simulink model "untitled1"  (R2022a)
settings: Solver=FixedStepAuto  StartTime=0.0  StopTime=10.0  RelTol=1e-3  EnableMultiTasking=on
settings Model: ExtModeTrigDuration=2  Creator=Asus  LastModifiedBy=Asus
settings OptimizationCC: EnhancedBackFolding=on  PassReuseOutputArgsAs=Individual arguments  ZeroExternalMemoryAtStartup=off  ZeroInternalMemoryAtStartup=off  MaxStackSize=64  OptimizeBlockOrder=speed  DifferentSizesBufferReuse=on  OptimizationCustomize=off  EfficientTunableParamExpr=on
settings DebuggingCC: ParameterTunabilityLossMsg=error
settings HardwareCC: ProdBitPerInt=16  ProdBitPerPointer=16  ProdBitPerSizeT=16  ProdBitPerPtrDiffT=16  ProdLargestAtomicFloat=None  ProdWordSize=8  ProdHWDeviceType=Atmel->AVR
settings SFSimCC: MATLABDynamicMemAlloc=off
settings RTWCC: SystemTargetFile=ert.tlc  HardwareBoard=Arduino Mega 2560  TemplateMakefile=ert_default_tmf  GenerateReport=on  Toolchain=Arduino AVR  BuildConfiguration=Faster Runs  LaunchReport=on
settings CodeAppCC: ForceParamTrailComments=on  IgnoreCustomStorageClasses=off  OperatorAnnotations=on  SimulinkDataObjDesc=on  SFDataObjDesc=on  InsertBlockDesc=on
settings ERTTargetCC: SupportContinuousTime=on  SupportVariableSizeSignals=on  ExtModeTransport=3  ExtModeStaticAlloc=on  ExtModeStaticAllocSize=2048  ExtModeMexFile=ext_xcp  ExtModeIntrfLevel=Level2 - Open

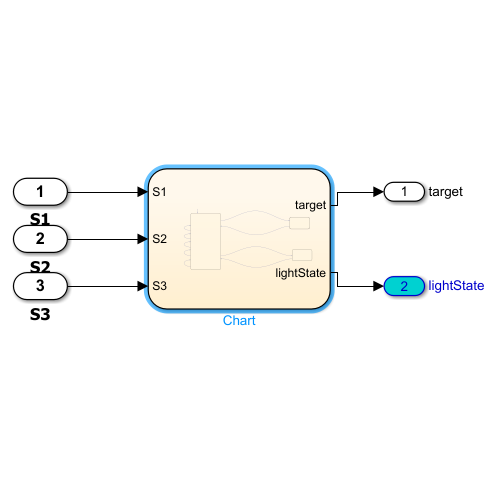
[thumbnail: Simulink's stored preview of the top-level diagram]
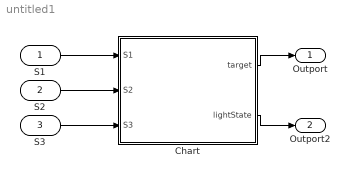
== system untitled1 ==
  S1 : Inport  OutDataTypeStr=boolean
  S2 : Inport  Port=2  OutDataTypeStr=boolean
  S3 : Inport  Port=3  OutDataTypeStr=boolean
  Chart : Stateflow chart  TreatAsAtomicUnit=on
  Outport : Outport  SignalName=target
  Outport2 : Outport  Port=2  SignalName=lightState
  wires:
  S2/1 -> Chart/2(S2)
  S3/1 -> Chart/3(S3)
  Chart/1(target) -> Outport/1
  Chart/2(lightState) -> Outport2/1
  S1/1 -> Chart/1(S1)

== stateflow chart untitled1/Chart ==
  state M
    entry:
    lightState=false;
    target=0;
  state SL2
    entry:
    target=2;
    lightState=true;
  state SL3
    entry:
    target=3;
    lightState=true;
  (default) -> M
  M -> SL2 [order 6] : [S1]
  M -> M [order 5] : [S2 && S3]
  SL2 -> M : [S2 || S3 || ~S1]
  M -> M [order 4] : [S1 && S3]
  M -> M [order 3] : [S1 && S2]
  M -> SL3 [order 7] : [S2]
  M -> M [order 2] : [S1 && S2 && S3]
  SL3 -> M : [S1 || S3 || ~S2]
  M -> M [order 1] : [~S1 && ~S2 && ~S3]
  data: target output int16; lightState output boolean; S1 input boolean; S2 input boolean; S3 input boolean
